simulink model "Worked_Example_2_3"  (R2024b)
settings: Solver=VariableStepAuto  StartTime=0.0  StopTime=20  RelTol=1e-3
settings Model: Creator=GH-X-ST  LastModifiedBy=GH-X-ST

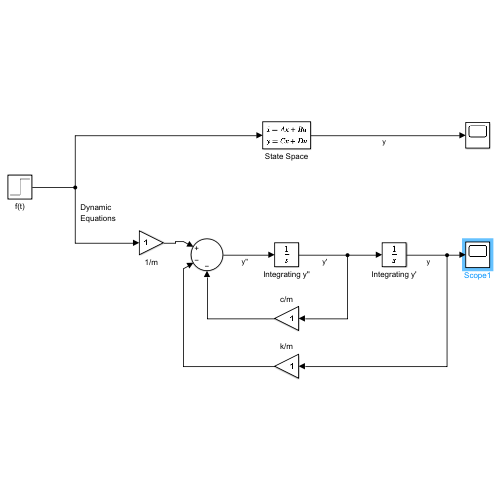
[thumbnail: Simulink's stored preview of the top-level diagram]
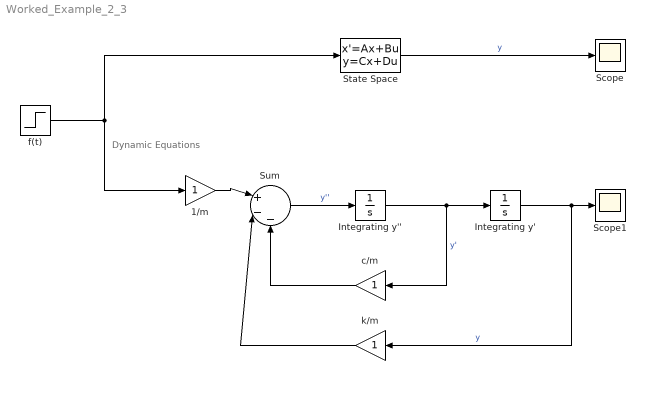
== system Worked_Example_2_3 ==
  note: Dynamic
      | Equations
  1/m : Gain
  Integrating y' : Integrator
  Integrating y'' : Integrator
  Scope : Scope
  Scope1 : Scope
  State Space : StateSpace  A=[0, 1; -1, -1]  B=[0; 1]  C=[1, 0]  D=[0]  InitialCondition=[0, 0]  ContinuousStateAttributes='position'
  Sum : Sum  Inputs=|+--
  c/m : Gain
  f(t) : Step  Time=0  SampleTime=0
  k/m : Gain
  wires:
  f(t)/1 -> State Space/1, 1/m/1
  State Space/1 -> Scope/1  "y"
  Integrating y''/1 -> c/m/1, Integrating y'/1  "y'"
  Integrating y'/1 -> Scope1/1, k/m/1  "y"
  1/m/1 -> Sum/1
  Sum/1 -> Integrating y''/1  "y''"
  c/m/1 -> Sum/3
  k/m/1 -> Sum/2
